simulink model "Controllo_Ottimo_LQ_Disturbi"  (R2023b)
settings: Solver=VariableStepAuto  StartTime=0.0  StopTime=50  RelTol=1e-3
undefined symbols (not defined in the file): A, A_obs, B, B_obs, C, C_obs, D, D_obs, Fi, Fr, Tc
libraries: simulink x2
settings Model: Creator=emman  LastModifiedBy=emman

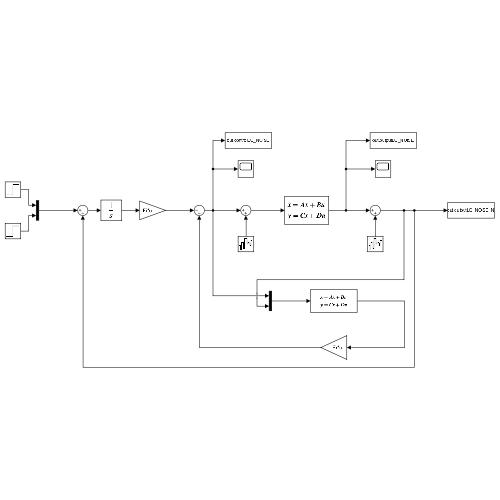
[thumbnail: Simulink's stored preview of the top-level diagram]
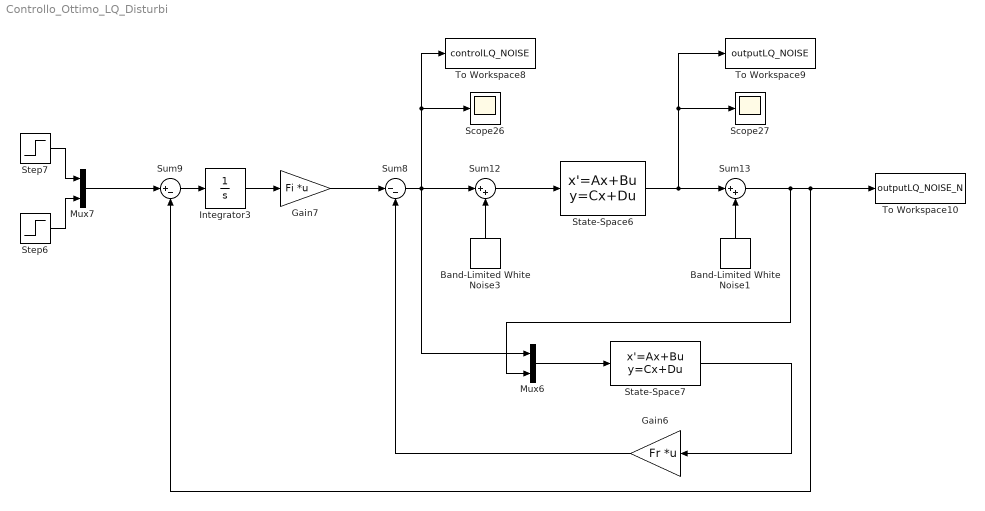
== system Controllo_Ottimo_LQ_Disturbi ==
  Band-Limited White Noise1 : simulink/Sources/Band-Limited White Noise  Cov=NoisePower  Ts=Tc  seed=[23341]
  Band-Limited White Noise3 : simulink/Sources/Band-Limited White Noise  Cov=Qnoise  Ts=Tc  seed=[23341]
  Gain6 : Gain  Gain=Fr  Multiplication=Matrix(K*u)
  Gain7 : Gain  Gain=Fi  Multiplication=Matrix(K*u)
  Integrator3 : Integrator
  Mux6 : Mux  Inputs=2
  Mux7 : Mux  Inputs=2
  Scope26 : Scope
  Scope27 : Scope
  State-Space6 : StateSpace  A=A  B=B  C=C  D=D  InitialCondition=0  ParameterTunability=Unconstrained
  State-Space7 : StateSpace  A=A_obs  B=B_obs  C=C_obs  D=D_obs  InitialCondition=0
  Step6 : Step  Time=0  After=2.5  SampleTime=0
  Step7 : Step  Time=0  After=2  SampleTime=0
  Sum12 : Sum  Inputs=|++
  Sum13 : Sum  Inputs=|++
  Sum8 : Sum  Inputs=|--
  Sum9 : Sum  Inputs=|+-
  To Workspace10 : ToWorkspace  VariableName=outputLQ_NOISE_N  SaveFormat=Structure With Time  SampleTime=-1
  To Workspace8 : ToWorkspace  VariableName=controlLQ_NOISE  SaveFormat=Structure With Time  SampleTime=-1
  To Workspace9 : ToWorkspace  VariableName=outputLQ_NOISE  SaveFormat=Structure With Time  SampleTime=-1
  wires:
  Sum12/1 -> State-Space6/1
  Band-Limited White Noise1/1 -> Sum13/2
  Band-Limited White Noise3/1 -> Sum12/2
  Sum8/1 -> Scope26/1, To Workspace8/1, Mux6/1, Sum12/1
  Sum13/1 -> Mux6/2, To Workspace10/1, Sum9/2
  State-Space6/1 -> Scope27/1, To Workspace9/1, Sum13/1
  State-Space7/1 -> Gain6/1
  Step6/1 -> Mux7/2
  Gain7/1 -> Sum8/1
  Mux6/1 -> State-Space7/1
  Gain6/1 -> Sum8/2
  Sum9/1 -> Integrator3/1
  Mux7/1 -> Sum9/1
  Integrator3/1 -> Gain7/1
  Step7/1 -> Mux7/1
